simulink model "test_binary"  (R2017b)
settings: Solver=FixedStepDiscrete  StartTime=0.0  StopTime=10.0  FixedStep=0.100000  RelTol=1e-3
model workspace (MAT data in the model file):
  already_pp = 1
settings Model: Creator=fconzelm  LastModifiedBy=hbourbou
settings DebuggingCC: AlgebraicLoopMsg=error  ArtificialAlgebraicLoopMsg=error  SingleTaskRateTransMsg=error

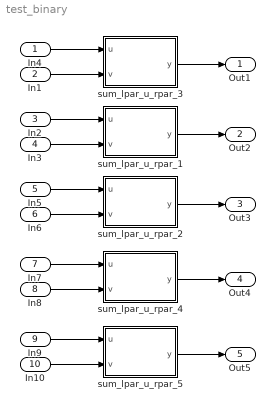
== system test_binary ==
  In4 : Inport  OutDataTypeStr=double  PortDimensions=[2 3]
  In1 : Inport  Port=2  OutDataTypeStr=double  PortDimensions=[2 3]
  In2 : Inport  Port=3  OutDataTypeStr=double  PortDimensions=[2 3]
  In3 : Inport  Port=4  OutDataTypeStr=double  PortDimensions=[2 3]
  In5 : Inport  Port=5  OutDataTypeStr=double  PortDimensions=[2 3]
  In6 : Inport  Port=6  OutDataTypeStr=double  PortDimensions=[2 3]
  In7 : Inport  Port=7  OutDataTypeStr=double  PortDimensions=[2 3]
  In8 : Inport  Port=8  OutDataTypeStr=double  PortDimensions=[2 3]
  In9 : Inport  Port=9  OutDataTypeStr=double  PortDimensions=[2 3]
  In10 : Inport  Port=10  OutDataTypeStr=double  PortDimensions=[2 3]
  sum_lpar_u_rpar_1 : MATLAB Function  TreatAsAtomicUnit=on
  sum_lpar_u_rpar_2 : MATLAB Function  TreatAsAtomicUnit=on
  sum_lpar_u_rpar_3 : MATLAB Function  TreatAsAtomicUnit=on
  sum_lpar_u_rpar_4 : MATLAB Function  TreatAsAtomicUnit=on
  sum_lpar_u_rpar_5 : MATLAB Function  TreatAsAtomicUnit=on
  Out1 : Outport
  Out2 : Outport  Port=2
  Out3 : Outport  Port=3
  Out4 : Outport  Port=4
  Out5 : Outport  Port=5
  wires:
  sum_lpar_u_rpar_3/1(y) -> Out1/1
  sum_lpar_u_rpar_1/1(y) -> Out2/1
  sum_lpar_u_rpar_2/1(y) -> Out3/1
  sum_lpar_u_rpar_4/1(y) -> Out4/1
  In1/1 -> sum_lpar_u_rpar_3/2(v)
  In4/1 -> sum_lpar_u_rpar_3/1(u)
  In2/1 -> sum_lpar_u_rpar_1/1(u)
  In5/1 -> sum_lpar_u_rpar_2/1(u)
  In7/1 -> sum_lpar_u_rpar_4/1(u)
  In9/1 -> sum_lpar_u_rpar_5/1(u)
  In8/1 -> sum_lpar_u_rpar_4/2(v)
  In6/1 -> sum_lpar_u_rpar_2/2(v)
  In3/1 -> sum_lpar_u_rpar_1/2(v)
  In10/1 -> sum_lpar_u_rpar_5/2(v)
  sum_lpar_u_rpar_5/1(y) -> Out5/1

== matlab function test_binary/sum_lpar_u_rpar_1 ==
  data: u input; y output; v input
function y = and1(u, v)

y = and(u, v);

== matlab function test_binary/sum_lpar_u_rpar_2 ==
  data: u input; y output; v input
function y = xor1(u, v)

y = xor(u, v);

== matlab function test_binary/sum_lpar_u_rpar_3 ==
  data: u input; y output; v input
function y = or1(u, v)

y = or(u, v);

== matlab function test_binary/sum_lpar_u_rpar_4 ==
  data: u input; y output; v input
function y = plus1(u, v)

y = plus(u, v);

== matlab function test_binary/sum_lpar_u_rpar_5 ==
  data: u input; y output; v input
function y = minus1(u, v)

y = minus(u, v);
